simulink model "W03_0_offline"  (R2024b)
settings: Solver=ode4  StartTime=0.0  StopTime=T_end_teleop  FixedStep=Ts  RelTol=1e-3
values from neighbouring files (symbols this model uses):
  animate = 1    [W03_setup.m]
  half_beam = 1.027135    [W03_setup.m]
  Izz = 653    [W03_setup.m]    (also in build_w03_models.m = p(2))
  m_usv = 211    [W03_setup.m]
  Nr = 800    [W03_setup.m]
  Nrr = 800    [W03_setup.m]    (also in build_w03_models.m = p(8))
  teleop_thrust = 200    [W03_setup.m]
  Ts = 0.05    [W03_setup.m]
  x0_w03 = zeros(6,1)    [W03_setup.m]
  Xu = 100    [W03_setup.m]    (also in build_w03_models.m = p(3))
  Xuu = 150    [W03_setup.m]    (also in build_w03_models.m = p(4))
  Yv = 100    [W03_setup.m]    (also in build_w03_models.m = p(5))
  Yvv = 100    [W03_setup.m]    (also in build_w03_models.m = p(6);'                newline  'Nr=p(7))
settings Model: Creator=admin  LastModifiedBy=admin

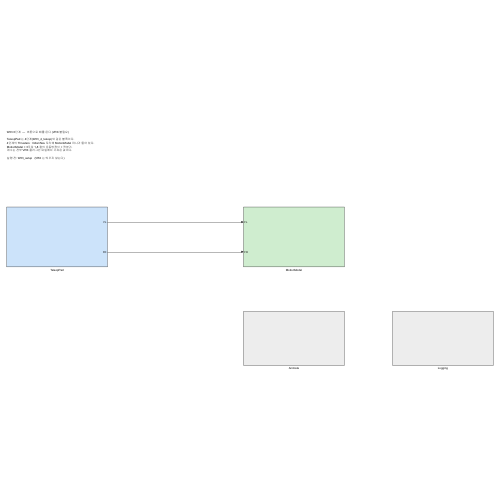
[thumbnail: Simulink's stored preview of the top-level diagram]
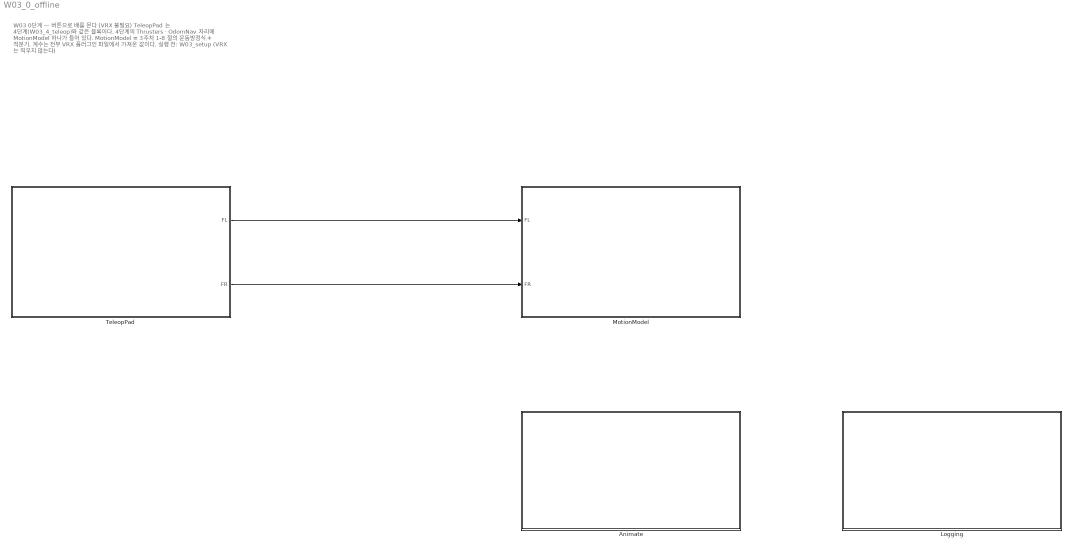
== system W03_0_offline ==
  note: W03 0단계  —  버튼으로 배를 몬다 (VRX 불필요)
      |
      | TeleopPad 는 4단계(W03_4_teleop)와 같은 블록이다.
      | 4단계의 Thrusters · OdomNav 자리에 MotionModel 하나가 들어 있다.
      | MotionModel = 3주차 1-8 절의 운동방정식 + 적분기.
      | 계수는 전부 VRX 플러그인 파일에서 가져온 값이다.
      |
      | 실행 전: W03_setup   (VRX 는 띄우지 않는다)
  Animate : Subsystem
  Logging : Subsystem
  MotionModel : Subsystem
  TeleopPad : Subsystem
  wires:
  TeleopPad/1(FL) -> MotionModel/1(FL)
  TeleopPad/2(FR) -> MotionModel/2(FR)

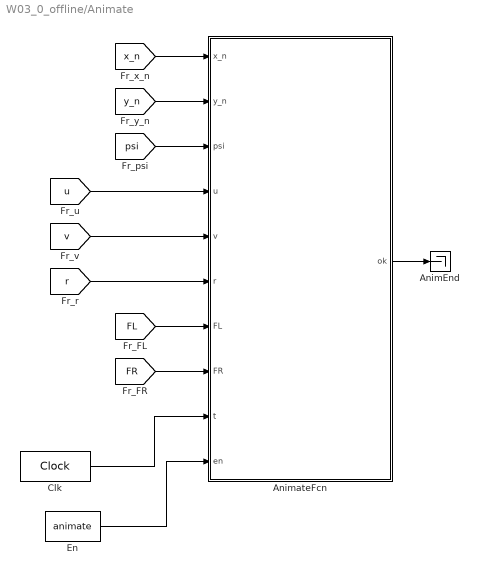
== system W03_0_offline/Animate ==
  AnimEnd : Terminator
  AnimateFcn : MATLAB Function  TreatAsAtomicUnit=on
  Clk : DigitalClock  SampleTime=Ts
  En : Constant  Value=animate
  wires:
  [v] -> AnimateFcn/5(v)
  En/1 -> AnimateFcn/10(en)
  Clk/1 -> AnimateFcn/9(t)
  [r] -> AnimateFcn/6(r)
  [u] -> AnimateFcn/4(u)
  AnimateFcn/1(ok) -> AnimEnd/1
  [FL] -> AnimateFcn/7(FL)
  [FR] -> AnimateFcn/8(FR)
  [psi] -> AnimateFcn/3(psi)
  [y_n] -> AnimateFcn/2(y_n)
  [x_n] -> AnimateFcn/1(x_n)

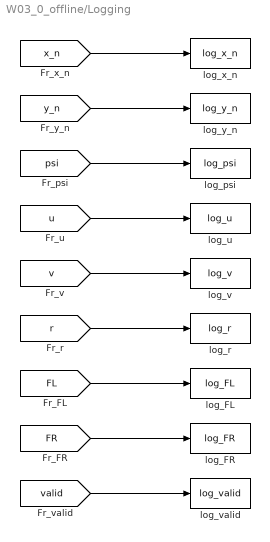
== system W03_0_offline/Logging ==
  log_FL : ToWorkspace  VariableName=log_FL  SaveFormat=Timeseries  SampleTime=Ts
  log_FR : ToWorkspace  VariableName=log_FR  SaveFormat=Timeseries  SampleTime=Ts
  log_psi : ToWorkspace  VariableName=log_psi  SaveFormat=Timeseries  SampleTime=Ts
  log_r : ToWorkspace  VariableName=log_r  SaveFormat=Timeseries  SampleTime=Ts
  log_u : ToWorkspace  VariableName=log_u  SaveFormat=Timeseries  SampleTime=Ts
  log_v : ToWorkspace  VariableName=log_v  SaveFormat=Timeseries  SampleTime=Ts
  log_valid : ToWorkspace  VariableName=log_valid  SaveFormat=Timeseries  SampleTime=Ts
  log_x_n : ToWorkspace  VariableName=log_x_n  SaveFormat=Timeseries  SampleTime=Ts
  log_y_n : ToWorkspace  VariableName=log_y_n  SaveFormat=Timeseries  SampleTime=Ts
  wires:
  [x_n] -> log_x_n/1
  [y_n] -> log_y_n/1
  [psi] -> log_psi/1
  [u] -> log_u/1
  [v] -> log_v/1
  [r] -> log_r/1
  [FL] -> log_FL/1
  [FR] -> log_FR/1
  [valid] -> log_valid/1

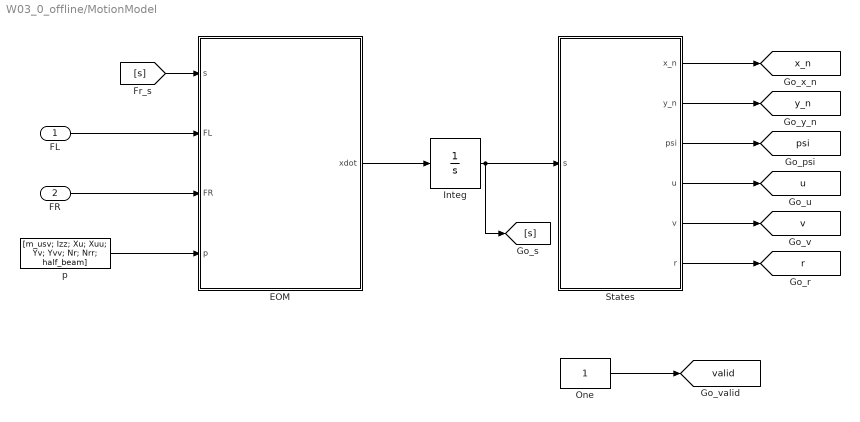
== system W03_0_offline/MotionModel ==
  FL : Inport
  FR : Inport  Port=2
  EOM : MATLAB Function  TreatAsAtomicUnit=on
  Integ : Integrator  InitialCondition=x0_w03
  One : Constant
  States : MATLAB Function  TreatAsAtomicUnit=on
  p : Constant  Value=[m_usv; Izz; Xu; Xuu; Yv; Yvv; Nr; Nrr; half_beam]
  tag scope: psi=global, r=global, u=global, v=global, valid=global, x_n=global, y_n=global
  wires:
  EOM/1(xdot) -> Integ/1
  Integ/1 -> States/1(s), [s]
  States/1(x_n) -> [x_n]
  States/2(y_n) -> [y_n]
  States/3(psi) -> [psi]
  States/4(u) -> [u]
  States/5(v) -> [v]
  States/6(r) -> [r]
  FL/1 -> EOM/2(FL)
  FR/1 -> EOM/3(FR)
  p/1 -> EOM/4(p)
  One/1 -> [valid]
  [s] -> EOM/1(s)

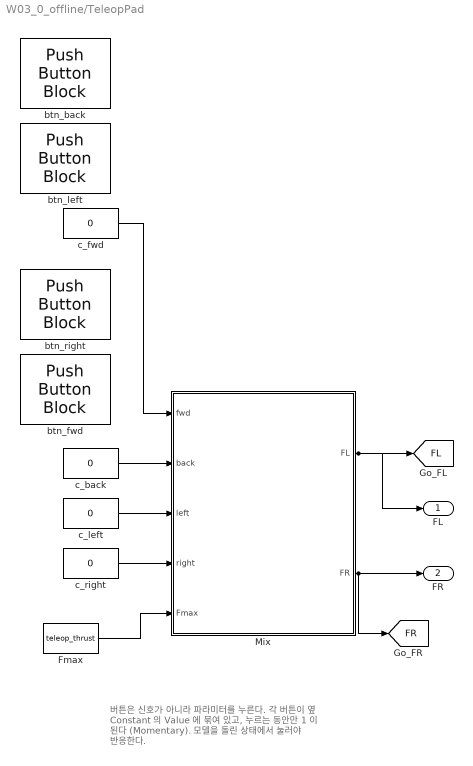
== system W03_0_offline/TeleopPad ==
  note: 버튼은 신호가 아니라 파라미터를 누른다.
      | 각 버튼이 옆 Constant 의 Value 에 묶여 있고,
      | 누르는 동안만 1 이 된다 (Momentary).
      | 모델을 돌린 상태에서 눌러야 반응한다.
  Fmax : Constant  Value=teleop_thrust
  Mix : MATLAB Function  TreatAsAtomicUnit=on
  btn_back : PushButtonBlock  ButtonText=▼ 후진
  btn_fwd : PushButtonBlock  ButtonText=▲ 전진
  btn_left : PushButtonBlock  ButtonText=◀ 좌선회
  btn_right : PushButtonBlock  ButtonText=▶ 우선회
  c_back : Constant  Value=0
  c_fwd : Constant  Value=0
  c_left : Constant  Value=0
  c_right : Constant  Value=0
  FL : Outport
  FR : Outport  Port=2
  tag scope: FL=global, FR=global
  wires:
  c_fwd/1 -> Mix/1(fwd)
  c_back/1 -> Mix/2(back)
  c_left/1 -> Mix/3(left)
  c_right/1 -> Mix/4(right)
  Fmax/1 -> Mix/5(Fmax)
  Mix/1(FL) -> [FL], FL/1
  Mix/2(FR) -> FR/1, [FR]

== matlab function W03_0_offline/MotionModel/EOM ==
  data: s input; xdot output; FL input; FR input; p input
function xdot = EOM(s, FL, FR, p)
%#codegen
% 3-DOF WAM-V equations of motion, NED.
% Coefficients come straight from the Gazebo VRX plugins.
%   s = [u v r x_n y_n psi]'
%   p = [m Izz Xu Xuu Yv Yvv Nr Nrr half_beam]'
u = s(1); v = s(2); r = s(3); psi = s(6);
m=p(1); Izz=p(2); Xu=p(3); Xuu=p(4); Yv=p(5); Yvv=p(6);
Nr=p(7); Nrr=p(8); b_half=p(9);

X = FL + FR;
N = (FL - FR)*b_half;

Dx = (Xu + Xuu*abs(u))*u;
Dy = (Yv + Yvv*abs(v))*v;
Dn = (Nr + Nrr*abs(r))*r;

du = (X - Dx)/m + v*r;
dv = (  - Dy)/m - u*r;
dr = (N - Dn)/Izz;

xdot = [du; dv; dr;
        u*cos(psi) - v*sin(psi);
        u*sin(psi) + v*cos(psi);
        r];

== matlab function W03_0_offline/TeleopPad/Mix ==
  data: fwd input; FL output; back input; left input; right input; Fmax input; FR output
function [FL, FR] = Mix(fwd, back, left, right, Fmax)
%#codegen
% wamv_teleop_key 와 같은 차동 배분.
%   전진   FL = +F, FR = +F      후진   FL = -F, FR = -F
%   좌선회 FL = -F, FR = +F      우선회 FL = +F, FR = -F
%
% 좌선회에서 요 모멘트 N = (FL - FR)*b 가 음수라 psi_NED 가 줄어든다.
surge = fwd   - back;
turn  = right - left;
FL = Fmax*(surge + turn);
FR = Fmax*(surge - turn);
FL = min(max(FL, -Fmax), Fmax);
FR = min(max(FR, -Fmax), Fmax);

== matlab function W03_0_offline/MotionModel/States ==
  data: s input; x_n output; y_n output; psi output; u output; v output; r output
function [x_n, y_n, psi, u, v, r] = States(s)
%#codegen
% 상태 벡터 s = [u v r x_n y_n psi] 에서 이름 있는 신호로 꺼낸다.
% psi 는 적분값이라 한 바퀴 돌면 2*pi 를 넘는다. OdomNav 와 같게 접는다.
u = s(1);  v = s(2);  r = s(3);
x_n = s(4);  y_n = s(5);
psi = atan2(sin(s(6)), cos(s(6)));

== matlab function W03_0_offline/Animate/AnimateFcn ==
  data: x_n input; y_n input; psi input; u input; ok output; v input; r input; FL input; FR input; t input; en input
function ok = AnimateFcn(x_n, y_n, psi, u, v, r, FL, FR, t, en)
%#codegen
% 그림은 코드 생성 대상이 아니므로 extrinsic 으로 부른다.
coder.extrinsic('W03_teleop_plot');
ok = 1;
if en > 0.5
    W03_teleop_plot(x_n, y_n, psi, u, v, r, FL, FR, t);
end
